simulink library "calcCLandCD"  (R2020a)
settings: Solver=VariableStepAuto  StartTime=0.0  StopTime=10.0  RelTol=1e-3
settings Model: Creator=Ayaz  LastModifiedBy=Ayaz

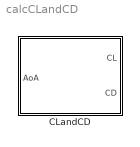
== system calcCLandCD ==
  CLandCD : Subsystem  mask{AoA_vals=0, CL_vals=0, CD_vals=0}
      mask prompts: AoA_vals "Angle of attack values [deg]"; CL_vals "Lift coeffcient values [-]"; CD_vals "Drag coefficient values [-]"

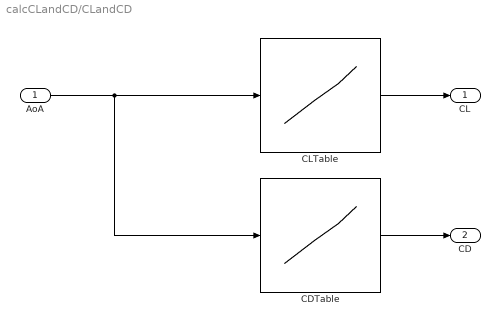
== system calcCLandCD/CLandCD ==
  AoA : Inport
  CDTable : Lookup_n-D  NumberOfTableDimensions=1  LookupTableObject=CLTable  BreakpointsForDimension1=AoA_vals  Table=CD_vals  DiagnosticForOutOfRangeInput=Warning  UseLastTableValue=on  InternalRulePriority=Speed  RndMeth=Simplest  InputSameDT=on
  CLTable : Lookup_n-D  NumberOfTableDimensions=1  LookupTableObject=CLTable  BreakpointsForDimension1=AoA_vals  Table=CL_vals  DiagnosticForOutOfRangeInput=Warning  UseLastTableValue=on  InternalRulePriority=Speed  RndMeth=Simplest  InputSameDT=on
  CL : Outport
  CD : Outport  Port=2
  wires:
  CDTable/1 -> CD/1
  CLTable/1 -> CL/1
  AoA/1 -> CDTable/1, CLTable/1
